simulink model "sm_abbYuMi_trajectory"  (R2021a)
settings: Solver=daessc  StartTime=0.0  StopTime=size(waypointsL, 2) * segment_duration  MaxStep=0.5  RelTol=1e-3  AbsTol=1e-3
values from neighbouring files (symbols this model uses):
  cube_l = 0.02    [startup_sm_abbYuMi_trajectory.m]
  segment_duration = 1.5    [sm_abbYuMi_trajectory_waypoints.m]    (also in startup_sm_abbYuMi_trajectory.m = 2)
undefined symbols (not defined in the file or in its folder): F1, F2, X, Y, Z
libraries: sm_lib x228, nesl_utility x52, robotcorelib x2
(part 6 of 6)

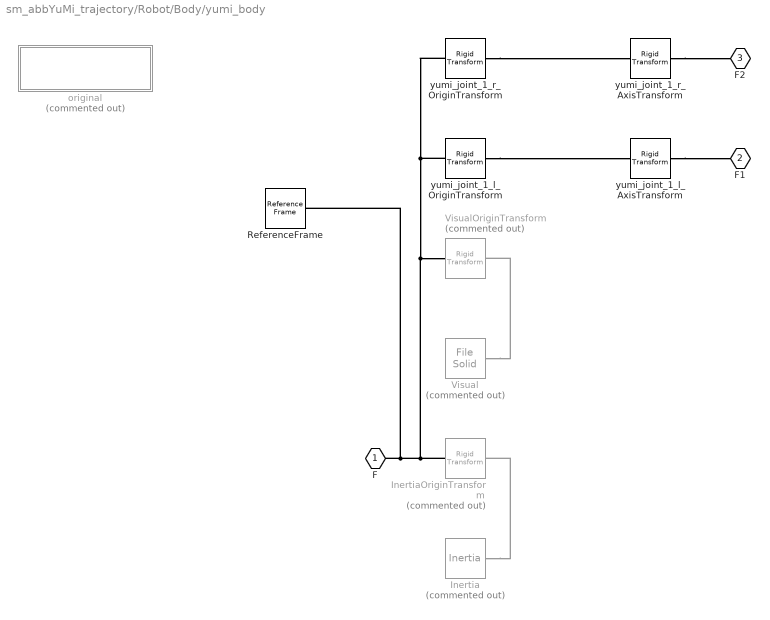
== system sm_abbYuMi_trajectory/Robot/Body/yumi_body ==
  Inertia : sm_lib/Body Elements/Inertia  Commented=on  InertiaType=Custom  Mass=15  MassUnits=kg  CenterOfMass=[0, 0, 0]  CenterOfMassUnits=m  MomentsOfInertia=[0.5, 0.6, 0.3]  MomentsOfInertiaUnits=kg*m^2  ProductsOfInertia=[0, 0, 0]  ProductsOfInertiaUnits=kg*m^2  GraphicType=None  MarkerShape=Inertia  MarkerSize=20  GraphicVisPropType=SimpleVisualProperties  GraphicDiffuseColor=[0.5 0.5 0.5]  GraphicSpecularColor=[0.5 0.5 0.5 1.0]  GraphicAmbientColor=[0.15 0.15 0.15 1.0]  GraphicEmissiveColor=[0.0 0.0 0.0 1.0]  GraphicShininess=75  GraphicOpacity=1.0
  InertiaOriginTransform : sm_lib/Frames and Transforms/Rigid Transform  Commented=on  TranslationMethod=Cartesian  TranslationStandardOffset=0  TranslationLengthUnit=m  TranslationStandardAxis=+Z  TranslationCartesianOffset=[0, 0, 0]  TranslationROffset=0  TranslationROffsetUnits=m  TranslationZOffset=0  TranslationZOffsetUnits=m  TranslationThetaOffset=0  TranslationThetaOffsetUnits=deg  RotationMethod=RotationSequence  RotationAngleUnits=deg  RotationStandardAxis=+Z  RotationAngle=0.0  RotationArbitraryAxis=[0 0 1]  FollAlignAxisA=+X  BaseAlignAxisA=+Y  FollAlignAxisB=+Y  BaseAlignAxisB=+Z  RotationSequenceAxes=BaseAxes  RotationSequence=XYZ  RotationSequenceAngles=[0, 0, 0]  RotationSequenceAnglesUnits=rad  RotationMatrix=[1 0 0; 0 1 0; 0 0 1]
  ReferenceFrame : sm_lib/Frames and Transforms/Reference Frame
  Visual : sm_lib/Body Elements/File Solid  Commented=on  ExtGeomFileName=abbyumi_body.stl  UnitType=Custom  ExtGeomFileUnits=m  StepReaderType=HEX  ExportConvexHullGeometry=off  InertiaType=Custom  Mass=0  MassUnits=kg  CenterOfMass=[0, 0, 0]  CenterOfMassUnits=m  MomentsOfInertia=[0, 0, 0]  MomentsOfInertiaUnits=kg*m^2  ProductsOfInertia=[0, 0, 0]  ProductsOfInertiaUnits=kg*m^2  BasedOnType=DensityFromFile  Density=1000  DensityUnits=kg/m^3  DoExposeReferenceFrame=on  SerializedFrames=<Frames/>  GraphicType=FromGeometry  MarkerShape=Sphere  MarkerSize=10  GraphicVisPropType=SimpleVisualProperties  GraphicDiffuseColor=[0.6 0.6 0.6]  GraphicSpecularColor=[0.5 0.5 0.5 1.0]  GraphicAmbientColor=[0.15 0.15 0.15 1.0]  GraphicEmissiveColor=[0.0 0.0 0.0 1.0]  GraphicShininess=75  GraphicOpacity=1
  VisualOriginTransform : sm_lib/Frames and Transforms/Rigid Transform  Commented=on  TranslationMethod=Cartesian  TranslationStandardOffset=0  TranslationLengthUnit=m  TranslationStandardAxis=+Z  TranslationCartesianOffset=[0, 0, 0]  TranslationROffset=0  TranslationROffsetUnits=m  TranslationZOffset=0  TranslationZOffsetUnits=m  TranslationThetaOffset=0  TranslationThetaOffsetUnits=deg  RotationMethod=RotationSequence  RotationAngleUnits=deg  RotationStandardAxis=+Z  RotationAngle=0.0  RotationArbitraryAxis=[0 0 1]  FollAlignAxisA=+X  BaseAlignAxisA=+Y  FollAlignAxisB=+Y  BaseAlignAxisB=+Z  RotationSequenceAxes=BaseAxes  RotationSequence=XYZ  RotationSequenceAngles=[0, 0, 0]  RotationSequenceAnglesUnits=rad  RotationMatrix=[1 0 0; 0 1 0; 0 0 1]
  original : Subsystem  Commented=on
  yumi_joint_1_l_AxisTransform : sm_lib/Frames and Transforms/Rigid Transform  TranslationMethod=Cartesian  TranslationStandardOffset=0  TranslationLengthUnit=m  TranslationStandardAxis=+Z  TranslationCartesianOffset=[0, 0, 0]  TranslationROffset=0  TranslationROffsetUnits=m  TranslationZOffset=0  TranslationZOffsetUnits=m  TranslationThetaOffset=0  TranslationThetaOffsetUnits=deg  RotationMethod=ArbitraryAxis  RotationAngleUnits=rad  RotationStandardAxis=+Z  RotationAngle=0  RotationArbitraryAxis=[1, 0, 0]  FollAlignAxisA=+X  BaseAlignAxisA=+Y  FollAlignAxisB=+Y  BaseAlignAxisB=+Z  RotationSequenceAxes=FollowerAxes  RotationSequence=XYX  RotationSequenceAngles=[0 0 0]  RotationSequenceAnglesUnits=deg  RotationMatrix=[1 0 0; 0 1 0; 0 0 1]
  yumi_joint_1_l_OriginTransform : sm_lib/Frames and Transforms/Rigid Transform  TranslationMethod=Cartesian  TranslationStandardOffset=0  TranslationLengthUnit=m  TranslationStandardAxis=+Z  TranslationCartesianOffset=[0, 0.6, 0]  TranslationROffset=0  TranslationROffsetUnits=m  TranslationZOffset=0  TranslationZOffsetUnits=m  TranslationThetaOffset=0  TranslationThetaOffsetUnits=deg  RotationMethod=StandardAxis  RotationAngleUnits=deg  RotationStandardAxis=+Z  RotationAngle=45  RotationArbitraryAxis=[0 0 1]  FollAlignAxisA=+X  BaseAlignAxisA=+Y  FollAlignAxisB=+Y  BaseAlignAxisB=+Z  RotationSequenceAxes=BaseAxes  RotationSequence=XYZ  RotationSequenceAngles=[0.9781, -0.5716, 2.318]  RotationSequenceAnglesUnits=rad  RotationMatrix=[1 0 0; 0 1 0; 0 0 1]
  yumi_joint_1_r_AxisTransform : sm_lib/Frames and Transforms/Rigid Transform  TranslationMethod=Cartesian  TranslationStandardOffset=0  TranslationLengthUnit=m  TranslationStandardAxis=+Z  TranslationCartesianOffset=[0, 0, 0]  TranslationROffset=0  TranslationROffsetUnits=m  TranslationZOffset=0  TranslationZOffsetUnits=m  TranslationThetaOffset=0  TranslationThetaOffsetUnits=deg  RotationMethod=ArbitraryAxis  RotationAngleUnits=rad  RotationStandardAxis=+Z  RotationAngle=0  RotationArbitraryAxis=[1, 0, 0]  FollAlignAxisA=+X  BaseAlignAxisA=+Y  FollAlignAxisB=+Y  BaseAlignAxisB=+Z  RotationSequenceAxes=FollowerAxes  RotationSequence=XYX  RotationSequenceAngles=[0 0 0]  RotationSequenceAnglesUnits=deg  RotationMatrix=[1 0 0; 0 1 0; 0 0 1]
  yumi_joint_1_r_OriginTransform : sm_lib/Frames and Transforms/Rigid Transform  TranslationMethod=Cartesian  TranslationStandardOffset=0  TranslationLengthUnit=m  TranslationStandardAxis=+Z  TranslationCartesianOffset=[0, -0.6, 0]  TranslationROffset=0  TranslationROffsetUnits=m  TranslationZOffset=0  TranslationZOffsetUnits=m  TranslationThetaOffset=0  TranslationThetaOffsetUnits=deg  RotationMethod=StandardAxis  RotationAngleUnits=deg  RotationStandardAxis=-Z  RotationAngle=45  RotationArbitraryAxis=[0 0 1]  FollAlignAxisA=+X  BaseAlignAxisA=+Y  FollAlignAxisB=+Y  BaseAlignAxisB=+Z  RotationSequenceAxes=BaseAxes  RotationSequence=XYZ  RotationSequenceAngles=[-0.9795, -0.5682, -2.3155]  RotationSequenceAnglesUnits=rad  RotationMatrix=[1 0 0; 0 1 0; 0 0 1]
  F : PMIOPort  Side=Left
  F1 : PMIOPort  Port=2  Side=Right
  F2 : PMIOPort  Port=3  Side=Right
  connections:
  Inertia/RConn1 -- InertiaOriginTransform/RConn1
  ReferenceFrame/RConn1 -- InertiaOriginTransform/LConn1 -- yumi_joint_1_l_OriginTransform/LConn1 -- yumi_joint_1_r_OriginTransform/LConn1 -- VisualOriginTransform/LConn1 -- F/RConn1
  Visual/RConn1 -- VisualOriginTransform/RConn1
  yumi_joint_1_l_AxisTransform/RConn1 -- F1/RConn1
  yumi_joint_1_r_AxisTransform/RConn1 -- F2/RConn1
  yumi_joint_1_r_OriginTransform/RConn1 -- yumi_joint_1_r_AxisTransform/LConn1
  yumi_joint_1_l_OriginTransform/RConn1 -- yumi_joint_1_l_AxisTransform/LConn1

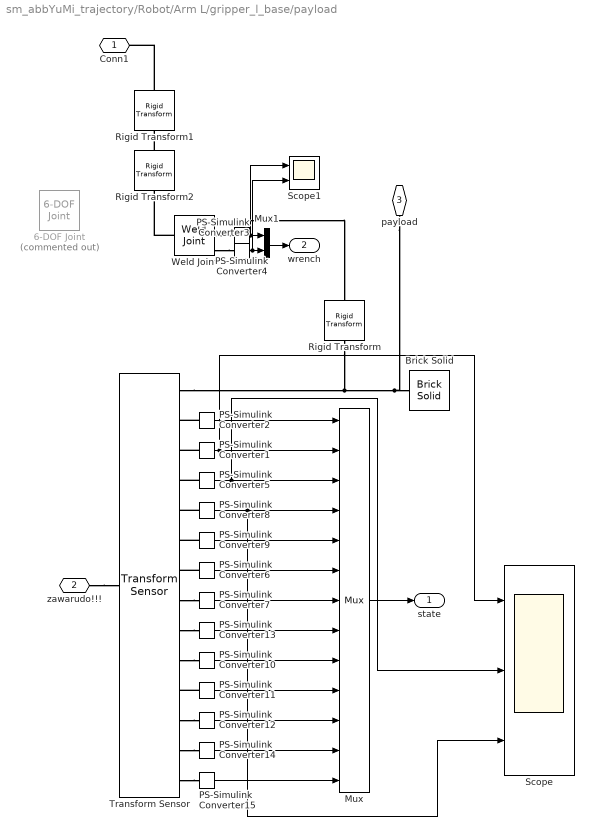
== system sm_abbYuMi_trajectory/Robot/Arm L/gripper_l_base/payload ==
  6-DOF Joint : sm_lib/Joints/6-DOF Joint  Commented=on  JointMode=Normal  SenseConstraintForce=off  SenseConstraintForceX=off  SenseConstraintForceY=off  SenseConstraintForceZ=off  SenseConstraintTorque=off  SenseConstraintTorqueX=off  SenseConstraintTorqueY=off  SenseConstraintTorqueZ=off  SenseTotalForce=on  SenseTotalForceX=off  SenseTotalForceY=off  SenseTotalForceZ=off  SenseTotalTorque=on  SenseTotalTorqueX=off  SenseTotalTorqueY=off  SenseTotalTorqueZ=off  CompositeWrenchDir=FollowerOnBase  CompositeWrenchFrame=BaseFrame  PxEquilibriumPosition=0  PxEquilibriumPositionUnits=m  PxSpringStiffness=0  PxSpringStiffnessUnits=N/m  PxDampingCoefficient=0  PxDampingCoefficientUnits=N/(m/s)  PxTorqueActuationMode=NoTorque  PxMotionActuationMode=ComputedMotion  PxSensePosition=off  PxSenseVelocity=off  PxSenseAcceleration=off  PxSenseTorqueForce=off  PxSenseLowerLimitTorqueForce=off  PxSenseUpperLimitTorqueForce=off  PxLowerLimitSpecify=on  PxLowerLimitBound=-0.05  PxLowerLimitBoundUnits=m  PxLowerLimitStiffness=1e2  PxLowerLimitStiffnessUnits=N/m  PxLowerLimitDamping=1e1  PxLowerLimitDampingUnits=N/(m/s)  PxLowerLimitTransitionRegionWidth=1e-4  PxLowerLimitTransitionRegionWidthUnits=m  PxUpperLimitSpecify=on  PxUpperLimitBound=0.05  PxUpperLimitBoundUnits=m  PxUpperLimitStiffness=1e2  PxUpperLimitStiffnessUnits=N/m  PxUpperLimitDamping=1e1  PxUpperLimitDampingUnits=N/(m/s)  PxUpperLimitTransitionRegionWidth=1e-4  PxUpperLimitTransitionRegionWidthUnits=m  PxPositionTargetSpecify=off  PxPositionTargetPriority=High  PxPositionTargetValue=0  PxPositionTargetValueUnits=m  PxVelocityTargetSpecify=off  PxVelocityTargetPriority=High  PxVelocityTargetValue=0  PxVelocityTargetValueUnits=m/s  PyEquilibriumPosition=0  PyEquilibriumPositionUnits=m  PySpringStiffness=0  PySpringStiffnessUnits=N/m  PyDampingCoefficient=0  PyDampingCoefficientUnits=N/(m/s)  PyTorqueActuationMode=NoTorque  PyMotionActuationMode=ComputedMotion  PySensePosition=off  PySenseVelocity=off  PySenseAcceleration=off  PySenseTorqueForce=off  PySenseLowerLimitTorqueForce=off  PySenseUpperLimitTorqueForce=off  PyLowerLimitSpecify=on  PyLowerLimitBound=-0.05  PyLowerLimitBoundUnits=m  PyLowerLimitStiffness=1e2  PyLowerLimitStiffnessUnits=N/m  PyLowerLimitDamping=1e1  PyLowerLimitDampingUnits=N/(m/s)  PyLowerLimitTransitionRegionWidth=1e-4  PyLowerLimitTransitionRegionWidthUnits=m  PyUpperLimitSpecify=on  PyUpperLimitBound=0.05  PyUpperLimitBoundUnits=m  PyUpperLimitStiffness=1e2  PyUpperLimitStiffnessUnits=N/m  PyUpperLimitDamping=1e1  PyUpperLimitDampingUnits=N/(m/s)  PyUpperLimitTransitionRegionWidth=1e-4  PyUpperLimitTransitionRegionWidthUnits=m  PyPositionTargetSpecify=off  PyPositionTargetPriority=High  PyPositionTargetValue=0  PyPositionTargetValueUnits=m  PyVelocityTargetSpecify=off  PyVelocityTargetPriority=High  PyVelocityTargetValue=0  PyVelocityTargetValueUnits=m/s  PzEquilibriumPosition=0  PzEquilibriumPositionUnits=m  PzSpringStiffness=0  PzSpringStiffnessUnits=N/m  PzDampingCoefficient=0  PzDampingCoefficientUnits=N/(m/s)  PzTorqueActuationMode=NoTorque  PzMotionActuationMode=ComputedMotion  PzSensePosition=off  PzSenseVelocity=off  PzSenseAcceleration=off  PzSenseTorqueForce=off  PzSenseLowerLimitTorqueForce=off  PzSenseUpperLimitTorqueForce=off  PzLowerLimitSpecify=on  PzLowerLimitBound=-0.01  PzLowerLimitBoundUnits=m  PzLowerLimitStiffness=1e2  PzLowerLimitStiffnessUnits=N/m  PzLowerLimitDamping=1e1  PzLowerLimitDampingUnits=N/(m/s)  PzLowerLimitTransitionRegionWidth=1e-4  PzLowerLimitTransitionRegionWidthUnits=m  PzUpperLimitSpecify=on  PzUpperLimitBound=0.05  PzUpperLimitBoundUnits=m  PzUpperLimitStiffness=1e2  PzUpperLimitStiffnessUnits=N/m  PzUpperLimitDamping=1e1  PzUpperLimitDampingUnits=N/(m/s)  PzUpperLimitTransitionRegionWidth=1e-4  PzUpperLimitTransitionRegionWidthUnits=m  PzPositionTargetSpecify=off  PzPositionTargetPriority=High  PzPositionTargetValue=0  PzPositionTargetValueUnits=m  PzVelocityTargetSpecify=off  PzVelocityTargetPriority=High  PzVelocityTargetValue=0  PzVelocityTargetValueUnits=m/s  SphDefPosRotationMethod=None  SphDefPosRotationAngleUnits=deg  SphDefPosRotationStandardAxis=+Z  SphDefPosRotationAngle=0.0  SphDefPosRotationArbitraryAxis=[0 0 1]  SphDefPosFollAlignAxisA=+X  SphDefPosBaseAlignAxisA=+Y  SphDefPosFollAlignAxisB=+Y  SphDefPosBaseAlignAxisB=+Z  SphDefPosRotationSequenceAxes=FollowerAxes  SphDefPosRotationSequence=XYX  SphDefPosRotationSequenceAngles=[0 0 0]  SphDefPosRotationSequenceAnglesUnits=deg  SphDefPosRotationMatrix=[1 0 0; 0 1 0; 0 0 1]  SphEqPosRotationMethod=None  SphEqPosRotationAngleUnits=deg  SphEqPosRotationStandardAxis=+Z  SphEqPosRotationAngle=0.0  SphEqPosRotationArbitraryAxis=[0 0 1]  SphEqPosFollAlignAxisA=+X  SphEqPosBaseAlignAxisA=+Y  SphEqPosFollAlignAxisB=+Y  SphEqPosBaseAlignAxisB=+Z  SphEqPosRotationSequenceAxes=FollowerAxes  SphEqPosRotationSequence=XYX  SphEqPosRotationSequenceAngles=[0 0 0]  SphEqPosRotationSequenceAnglesUnits=deg  SphEqPosRotationMatrix=[1 0 0; 0 1 0; 0 0 1]  SphSpringStiffness=0  SphSpringStiffnessUnits=N*m/deg  SphDampingCoefficient=0  SphDampingCoefficientUnits=N*m/(deg/s)  SphActuateTorqueX=off  SphActuateTorqueY=off  SphActuateTorqueZ=off  SphActuateTorque=off  SphTorqueActuationMode=NoTorque  SphMotionActuationMode=ComputedMotion  SphActuationFrame=BaseFrame  SphSensePosition=off  SphSenseVelocityX=off  SphSenseVelocityY=off  SphSenseVelocityZ=off  SphSenseVelocity=off  SphSenseAccelerationX=off  SphSenseAccelerationY=off  SphSenseAccelerationZ=off  SphSenseAcceleration=off  SphSenseTorqueX=off  SphSenseTorqueY=off  SphSenseTorqueZ=off  SphSenseTorqueForce=off  SphSenseLowerLimitTorqueMag=off  SphSenseUpperLimitTorqueMag=off  SphSensingFrame=BaseFrame  SphLowerLimitSpecify=on  SphLowerLimitBound=-15  SphLowerLimitBoundUnits=deg  SphLowerLimitStiffness=1e1  SphLowerLimitStiffnessUnits=N*m/deg  SphLowerLimitDamping=1  SphLowerLimitDampingUnits=N*m/(deg/s)  SphLowerLimitTransitionRegionWidth=0.1  SphLowerLimitTransitionRegionWidthUnits=deg  SphUpperLimitSpecify=on  SphUpperLimitBound=15  SphUpperLimitBoundUnits=deg  SphUpperLimitStiffness=1e1  SphUpperLimitStiffnessUnits=N*m/deg  SphUpperLimitDamping=1  SphUpperLimitDampingUnits=N*m/(deg/s)  SphUpperLimitTransitionRegionWidth=0.1  SphUpperLimitTransitionRegionWidthUnits=deg  SphPositionTargetRotationMethod=None  SphPositionTargetRotationAngleUnits=deg  SphPositionTargetRotationStandardAxis=+Z  SphPositionTargetRotationAngle=0.0  SphPositionTargetRotationArbitraryAxis=[0 0 1]  SphPositionTargetFollAlignAxisA=+X  SphPositionTargetBaseAlignAxisA=+Y  SphPositionTargetFollAlignAxisB=+Y  SphPositionTargetBaseAlignAxisB=+Z  SphPositionTargetRotationSequenceAxes=FollowerAxes  SphPositionTargetRotationSequence=XYX  SphPositionTargetRotationSequenceAngles=[0 0 0]  SphPositionTargetRotationSequenceAnglesUnits=deg  SphPositionTargetRotationMatrix=[1 0 0; 0 1 0; 0 0 1]  SphPositionTargetSpecify=off  SphPositionTargetPriority=High  SphVelocityTargetValue=[0 0 0]  SphVelocityTargetValueUnits=deg/s  SphVelocityTargetSpecify=off  SphVelocityTargetPriority=High  SphVelocityTargetInFollowerFrame=on
  Brick Solid : sm_lib/Body Elements/Brick Solid  GraphicAmbientColor=[0.15 0.15 0.15 1.0]  BasedOnType=Mass  BrickDimensions=[0.1 0.35 0.1]  BrickDimensionUnits=m  CenterOfMass=[0 0 0]  CenterOfMassUnits=m  GraphicDiffuseColor=[0.5 0.5 0.5]  Density=1000  DensityUnits=kg/m^3  DoExposeReferenceFrame=on  GraphicEmissiveColor=[0.0 0.0 0.0 1.0]  ExportEntireGeometry=off  SerializedFrames=<Frames/>  MarkerShape=Sphere  MarkerSize=10  GraphicType=FromGeometry  InertiaType=CalculateFromGeometry  Mass=1  MassUnits=kg  MomentsOfInertia=[1 1 1]  MomentsOfInertiaUnits=kg*m^2  GraphicOpacity=1.0  ProductsOfInertia=[0 0 0]  ProductsOfInertiaUnits=kg*m^2  GraphicShininess=75  GraphicSpecularColor=[0.5 0.5 0.5 1.0]  GraphicVisPropType=SimpleVisualProperties
  Mux : Mux  Inputs=13
  Mux1 : Mux  Inputs=2
  PS-Simulink Converter{1..15} (15 alike) : nesl_utility/PS-Simulink Converter  PhysicalDomain=network_engine_domain  SubClassName=ps_output  LeftPortType=input  RightPortType=output  PseudoPeriodic=off  Frequencies=[]  Unit=inherit  AffineConversion=off
      settings: SourceProductBaseCode=PW,SS
  Rigid Transform : sm_lib/Frames and Transforms/Rigid Transform  TranslationMethod=Cartesian  TranslationStandardOffset=0  TranslationLengthUnit=m  TranslationStandardAxis=+Z  TranslationCartesianOffset=[0 -0.175 0]  TranslationROffset=0  TranslationROffsetUnits=m  TranslationZOffset=0  TranslationZOffsetUnits=m  TranslationThetaOffset=0  TranslationThetaOffsetUnits=deg  RotationMethod=None  RotationAngleUnits=deg  RotationStandardAxis=+Z  RotationAngle=0.0  RotationArbitraryAxis=[0 0 1]  FollAlignAxisA=+X  BaseAlignAxisA=+Y  FollAlignAxisB=+Y  BaseAlignAxisB=+Z  RotationSequenceAxes=FollowerAxes  RotationSequence=XYX  RotationSequenceAngles=[0 0 0]  RotationSequenceAnglesUnits=deg  RotationMatrix=[1 0 0; 0 1 0; 0 0 1]
  Rigid Transform1 : sm_lib/Frames and Transforms/Rigid Transform  TranslationMethod=Cartesian  TranslationStandardOffset=0  TranslationLengthUnit=m  TranslationStandardAxis=+Z  TranslationCartesianOffset=[0 0 0.0837]  TranslationROffset=0  TranslationROffsetUnits=m  TranslationZOffset=0  TranslationZOffsetUnits=m  TranslationThetaOffset=0  TranslationThetaOffsetUnits=deg  RotationMethod=None  RotationAngleUnits=deg  RotationStandardAxis=+Z  RotationAngle=0.0  RotationArbitraryAxis=[0 0 1]  FollAlignAxisA=+X  BaseAlignAxisA=+Y  FollAlignAxisB=+Y  BaseAlignAxisB=+Z  RotationSequenceAxes=FollowerAxes  RotationSequence=XYX  RotationSequenceAngles=[0 0 0]  RotationSequenceAnglesUnits=deg  RotationMatrix=[1 0 0; 0 1 0; 0 0 1]
  Rigid Transform2 : sm_lib/Frames and Transforms/Rigid Transform  TranslationMethod=None  TranslationStandardOffset=0  TranslationLengthUnit=m  TranslationStandardAxis=+Z  TranslationCartesianOffset=[0 0 0.0837]  TranslationROffset=0  TranslationROffsetUnits=m  TranslationZOffset=0  TranslationZOffsetUnits=m  TranslationThetaOffset=0  TranslationThetaOffsetUnits=deg  RotationMethod=RotationSequence  RotationAngleUnits=deg  RotationStandardAxis=+Z  RotationAngle=0.0  RotationArbitraryAxis=[0 0 1]  FollAlignAxisA=+X  BaseAlignAxisA=+Y  FollAlignAxisB=+Y  BaseAlignAxisB=+Z  RotationSequenceAxes=FollowerAxes  RotationSequence=XYX  RotationSequenceAngles=[-90 -90 0]  RotationSequenceAnglesUnits=deg  RotationMatrix=[1 0 0; 0 1 0; 0 0 1]
  Scope : Scope  NumInputPorts=3
  Scope1 : Scope  NumInputPorts=2
  Transform Sensor : sm_lib/Frames and Transforms/Transform Sensor  MeasurementFrame=Base  SenseAngle=off  SenseAxis=off  SenseAngle1=off  SenseAngle2=off  SenseAngle3=off  SenseQ=on  SenseR=off  SenseOmegaX=on  SenseOmegaY=on  SenseOmegaZ=on  SenseOmega1=off  SenseOmega2=off  SenseOmega3=off  SenseQDot=off  SenseRDot=off  SenseAlphaX=off  SenseAlphaY=off  SenseAlphaZ=off  SenseAlpha1=off  SenseAlpha2=off  SenseAlpha3=off  SenseQDDot=off  SenseRDDot=off  SenseX=on  SenseY=on  SenseZ=on  SenseRad=off  SenseAzim=off  SenseDist=off  SenseInc=off  SenseXDot=on  SenseYDot=on  SenseZDot=on  SenseRadDot=off  SenseAzimDot=off  SenseDistDot=off  SenseIncDot=off  SenseXDDot=on  SenseYDDot=on  SenseZDDot=on  SenseRadDDot=off  SenseAzimDDot=off  SenseDistDDot=off  SenseIncDDot=off
  Weld Joint : sm_lib/Joints/Weld Joint  JointMode=Normal  SenseConstraintForce=off  SenseConstraintForceX=off  SenseConstraintForceY=off  SenseConstraintForceZ=off  SenseConstraintTorque=off  SenseConstraintTorqueX=off  SenseConstraintTorqueY=off  SenseConstraintTorqueZ=off  SenseTotalForce=on  SenseTotalForceX=off  SenseTotalForceY=off  SenseTotalForceZ=off  SenseTotalTorque=on  SenseTotalTorqueX=off  SenseTotalTorqueY=off  SenseTotalTorqueZ=off  CompositeWrenchDir=BaseOnFollower  CompositeWrenchFrame=FollowerFrame
  Conn1 : PMIOPort  Side=Left
  zawarudo!!! : PMIOPort  Port=2  Side=Left
  payload : PMIOPort  Port=3  Side=Right
  state : Outport
  wrench : Outport  Port=2
  wires:
  PS-Simulink Converter9/1 -> Mux/5
  PS-Simulink Converter2/1 -> Mux/1
  PS-Simulink Converter11/1 -> Mux/10
  PS-Simulink Converter10/1 -> Mux/9
  PS-Simulink Converter1/1 -> Scope/1, Mux/2
  PS-Simulink Converter13/1 -> Mux/8
  Mux/1 -> state/1
  PS-Simulink Converter7/1 -> Mux/7
  PS-Simulink Converter6/1 -> Mux/6
  PS-Simulink Converter5/1 -> Scope/2, Mux/3
  PS-Simulink Converter8/1 -> Scope/3, Mux/4
  Mux1/1 -> wrench/1
  PS-Simulink Converter4/1 -> Scope1/1, Mux1/1
  PS-Simulink Converter3/1 -> Scope1/2, Mux1/2
  PS-Simulink Converter12/1 -> Mux/11
  PS-Simulink Converter14/1 -> Mux/12
  PS-Simulink Converter15/1 -> Mux/13
  connections:
  Rigid Transform1/LConn1 -- Conn1/RConn1
  Weld Joint/RConn1 -- Rigid Transform/LConn1
  Rigid Transform/RConn1 -- Transform Sensor/RConn1 -- payload/RConn1 -- Brick Solid/RConn1
  Rigid Transform2/LConn1 -- Rigid Transform1/RConn1
  Weld Joint/LConn1 -- Rigid Transform2/RConn1
  PS-Simulink Converter1/LConn1 -- Transform Sensor/RConn3
  PS-Simulink Converter5/LConn1 -- Transform Sensor/RConn4
  Transform Sensor/RConn10 -- PS-Simulink Converter10/LConn1
  Transform Sensor/RConn9 -- PS-Simulink Converter13/LConn1
  PS-Simulink Converter2/LConn1 -- Transform Sensor/RConn2
  PS-Simulink Converter8/LConn1 -- Transform Sensor/RConn5
  PS-Simulink Converter6/LConn1 -- Transform Sensor/RConn7
  PS-Simulink Converter9/LConn1 -- Transform Sensor/RConn6
  PS-Simulink Converter11/LConn1 -- Transform Sensor/RConn11
  Transform Sensor/RConn8 -- PS-Simulink Converter7/LConn1
  zawarudo!!!/RConn1 -- Transform Sensor/LConn1
  Weld Joint/RConn2 -- PS-Simulink Converter4/LConn1
  Weld Joint/RConn3 -- PS-Simulink Converter3/LConn1
  Transform Sensor/RConn12 -- PS-Simulink Converter12/LConn1
  Transform Sensor/RConn13 -- PS-Simulink Converter14/LConn1
  Transform Sensor/RConn14 -- PS-Simulink Converter15/LConn1

== system sm_abbYuMi_trajectory/Robot/Body/yumi_body/original ==
  yumi_joint_1_l_OriginTransform : sm_lib/Frames and Transforms/Rigid Transform  TranslationMethod=Cartesian  TranslationStandardOffset=0  TranslationLengthUnit=m  TranslationStandardAxis=+Z  TranslationCartesianOffset=[0.05355, 0.0725, 0.41492]  TranslationROffset=0  TranslationROffsetUnits=m  TranslationZOffset=0  TranslationZOffsetUnits=m  TranslationThetaOffset=0  TranslationThetaOffsetUnits=deg  RotationMethod=RotationSequence  RotationAngleUnits=deg  RotationStandardAxis=+Z  RotationAngle=0.0  RotationArbitraryAxis=[0 0 1]  FollAlignAxisA=+X  BaseAlignAxisA=+Y  FollAlignAxisB=+Y  BaseAlignAxisB=+Z  RotationSequenceAxes=BaseAxes  RotationSequence=XYZ  RotationSequenceAngles=[0.9781, -0.5716, 2.318]  RotationSequenceAnglesUnits=rad  RotationMatrix=[1 0 0; 0 1 0; 0 0 1]
  yumi_joint_1_r_OriginTransform : sm_lib/Frames and Transforms/Rigid Transform  TranslationMethod=Cartesian  TranslationStandardOffset=0  TranslationLengthUnit=m  TranslationStandardAxis=+Z  TranslationCartesianOffset=[0.05355, -0.0725, 0.41492]  TranslationROffset=0  TranslationROffsetUnits=m  TranslationZOffset=0  TranslationZOffsetUnits=m  TranslationThetaOffset=0  TranslationThetaOffsetUnits=deg  RotationMethod=RotationSequence  RotationAngleUnits=deg  RotationStandardAxis=+Z  RotationAngle=0.0  RotationArbitraryAxis=[0 0 1]  FollAlignAxisA=+X  BaseAlignAxisA=+Y  FollAlignAxisB=+Y  BaseAlignAxisB=+Z  RotationSequenceAxes=BaseAxes  RotationSequence=XYZ  RotationSequenceAngles=[-0.9795, -0.5682, -2.3155]  RotationSequenceAnglesUnits=rad  RotationMatrix=[1 0 0; 0 1 0; 0 0 1]
  Conn1 : PMIOPort  Side=Left
  Conn2 : PMIOPort  Port=2  Side=Right
  Conn3 : PMIOPort  Port=3  Side=Left
  Conn4 : PMIOPort  Port=4  Side=Right
  connections:
  yumi_joint_1_r_OriginTransform/RConn1 -- Conn2/RConn1
  yumi_joint_1_l_OriginTransform/LConn1 -- Conn3/RConn1
  yumi_joint_1_l_OriginTransform/RConn1 -- Conn4/RConn1
  yumi_joint_1_r_OriginTransform/LConn1 -- Conn1/RConn1

== matlab function sm_abbYuMi_trajectory/observer/controller ==
  settings: updateMethod=DISCRETE  sampleTime=0.005
  data: y output; state input; wrench_b input; t input; aa output; b output; c output; dbg output; dbg1 output; dbg2 output; dbg3 output; dbg4 output
function [y,aa, b, c, dbg, dbg1, dbg2, dbg3, dbg4] = fcn(state, wrench_b, t)
%% gains
% ICL gain
N_o = 50;
ICL_switcher = true;
k_cl_m = 10;
k_cl_rp = 3;
k_cl_I = 1;
k_cl_Ixx = 30;
k_cl_Iyy = 120;
k_cl_Izz = 150;
k_cl_ri = 20;
k_cl = [k_cl_m k_cl_rp*ones(1,3) k_cl_Ixx k_cl_I k_cl_I k_cl_Iyy k_cl_I k_cl_Izz k_cl_ri*ones(1,3)];
k_cl_gain = diag(k_cl);

% gamma o
g_m = 1;
g_rp = 1;
g_I = 1;
g_ri = 1;
gg = [g_m g_rp*ones(1,3) g_I*ones(1,6) g_ri*ones(1,3)];
g_o = diag(gg);

% Kd matrix
Kdl = 0.001;
Kdr = 0.001;
Kdd = [Kdl*ones(1,3) Kdr*ones(1,3)];
Kd = diag(Kdd);

% sliding parameter
lambda = 1.5;

% deadband in which to stop adaptation
deadband = 0.00;

% robot number
N = 1;

%% function definition
function output = vee(matrix)
    output = [matrix(3, 2); matrix(1, 3); matrix(2, 1)];
end

function output = Pa(matrix)
    output = 0.5 * (matrix - matrix.');
end

function output = skew(v)
   output =  [    0 -v(3)   v(2)
               v(3)     0  -v(1)
              -v(2)  v(1)      0];
end

function output = L(v)
    output = [v(1)  v(2)  v(3)     0     0     0
                 0  v(1)     0  v(2)  v(3)     0
                 0     0  v(1)     0  v(2)  v(3)];
end
%% initialize
persistent v_last;
persistent w_last;
persistent index;
persistent mat_matrix;
persistent theta_o_hat;
persistent theta_o;
persistent Rd;
persistent xd;
persistent ICL_update;
persistent t_last;

if isempty(index)
        % ground truth
        mass = 1;
        center_of_mass = [0 0 0];
        inertia_matrix = [0.00833333, 0, 0, 0.00166667, 0, 0.00833333];
        r = [0 0.15 0];
        theta_o = [mass mass*center_of_mass inertia_matrix r].';
        
        % initial guess
        theta_o_hat = zeros(10 + 3 * N, 1);
        theta_o_hat = theta_o;
        % mass
        theta_o_hat(1) = 0;
        % COG
        theta_o_hat(2) = 0;
        theta_o_hat(3) = 0;
        theta_o_hat(4) = 0;
        % Inertia
        theta_o_hat(5) = 0.0;
        theta_o_hat(6) = 0.0;
        theta_o_hat(7) = 0.0;
        theta_o_hat(8) = 0.0;
        theta_o_hat(9) = 0.0;
        theta_o_hat(10) = 0.0;
        % grasp point
        theta_o_hat(11) = 0;
        theta_o_hat(12) = 0;
        theta_o_hat(13) = 0;
        
        % without ICL first time
        ICL_update = false;

        Rd = [1  0  0;
              0  1  0;
              0  0  1];

        xd = [0.27865; 0; 0.203];
        index = 1;
        v_last = zeros(3, 1);
        w_last = zeros(3, 1);
        mat_matrix = zeros(size(theta_o_hat, 1), N_o);
        t_last = 0;
end

mat_sum = zeros(size(theta_o_hat, 1), 1);
debug_msg = zeros(6, 1);
dt = t - t_last;
G = [0; 0; -9.80665];

%% unpack ref
% vd = [ref(1); ref(2); ref(3)];
% wd = [ref(4); ref(5); ref(6)];
% ad = [ref(7); ref(8); ref(9)];
% ald = [ref(10); ref(11); ref(12)];

%% unpack state
quat = [state(1) state(2) state(3) state(4)];
R = quat2rotm(quat);
w = [state(5); state(6); state(7)];
x = [state(8); state(9); state(10)];
v = [state(11); state(12); state(13)];
a = [state(14); state(15); state(16)];

wrench = [         R, zeros(3,3);
          zeros(3,3),          R] * wrench_b;
force = [wrench(1); wrench(2); wrench(3)];

%% compute error signals
% Re = Rd.' * R;
% we = w - wd;

%% compute composite error s
% sigma = we + lambda * Rd * vee(Pa(Re));
% v_t = v - vd;
% x_t = x - xd;
% s = [v_t + lambda * x_t;
%                   sigma];

%% regression matrix
% alpha_r = ald - lambda * skew(wd) * Rd * vee(Pa(Re)) - lambda * Rd * vee(Pa(skew(Rd.' * we) * Re));
% w_r = wd - lambda * Rd * vee(Pa(Re));
% a_r = ad - lambda * v_t;
% v_r = vd - lambda * x_t;
% 
% Y_l = [a_r, -skew(alpha_r) * R - skew(w) * skew(w_r) * R, zeros(3,6+3*N)];
% Y_r = [zeros(3,1), skew(a_r) * R + skew(w) * skew(v_r) * R - skew(w_r) * skew(v) * R, R * L(R.' * alpha_r) + skew(w) * R * L(R.' * w_r), skew(force)*R];
% % for i=1:N
% %     Y_r = [Y_r skew(force)*R];
% % end
% Y_o = [Y_l;
%        Y_r];
   
%% ICL
if ICL_update && ICL_switcher
    y_l = [(a - G) * dt, -skew(w - w_last) * R - (skew(w) * skew(w) * R) * dt, zeros(3,6 + 3 * N)];
    y_r = [zeros(3,1), skew(a - G) * R * dt, R * L(R.' * (w - w_last)) + (skew(w) * R * L(R.' * w)) * dt, skew(force) * R * dt];
%       y_l = [v - v_last, -skew(w - w_last) * R - (skew(w) * skew(w) * R) * dt, zeros(3,6 + 3 * N)];
%       y_r = [zeros(3,1), skew(v - v_last) * R, R * L(R.' * (w - w_last)) + (skew(w) * R * L(R.' * w)) * dt, skew(force) * R * dt];
%     for i = 1:N
%         y_r = hcat(y_r, skew(force[i])*R*dt)
%     end
    y_o_cl_integral = [y_l;
                       y_r];

    if index > N_o
        index = 1;
    end

    true_tau_integral = zeros(6, 1);
    for i = 1:N
        true_tau_integral = true_tau_integral + wrench * dt;
    end
    y_o_cl_integral_a_hat = y_o_cl_integral * theta_o_hat;
    mat_now = y_o_cl_integral.' * (y_o_cl_integral_a_hat - true_tau_integral);
    
    
    debug_msg = y_o_cl_integral * theta_o - true_tau_integral;

    
    mat_matrix(:, index) = mat_now;

    mat_sum = sum(mat_matrix, 2);

    index = index + 1;

    v_last = v;
    w_last = w;
    t_last = t;
end

theta_o_hat_dot = zeros(10 + 3 * N, 1);
if ICL_update && ICL_switcher
%     theta_o_hat_dot = -g_o * Y_o.' * s - k_cl_gain * g_o * mat_sum;
    theta_o_hat_dot = - k_cl_gain * g_o * mat_sum;
% else
%     theta_o_hat_dot = -g_o * Y_o.' * s;
end

% decide whether update or not
% if norm(s) < deadband
%     ICL_update = false;
% else
%     ICL_update = true;
% end
ICL_update = true;
%% desired signal calculate
% Rd = exp(dt * skew(wd)) .* Rd;
% xd = xd + v * dt + 0.5 * ad * dt * dt;

%% update law
theta_o_hat = theta_o_hat + theta_o_hat_dot * dt;

%% controller
% tau = -Kd * s + Y_o * theta_o_hat;

%% debug


%% output
y = 0;
aa = theta_o_hat(1:4);
b = theta_o_hat(5:10);
c = theta_o_hat(11:13);
dbg = theta_o_hat;
dbg1 = R;
dbg2 = dt;
dbg3 = v;
dbg4 = 0;
end
